simulink model "mat_ffun"  (R2015b)
settings: Solver=VariableStepAuto  StartTime=0.0  StopTime=100  RelTol=1e-3
undefined symbols (not defined in the file): alpha, delta_e, V, w
settings Model: Creator=Pramod  LastModifiedBy=Pramod

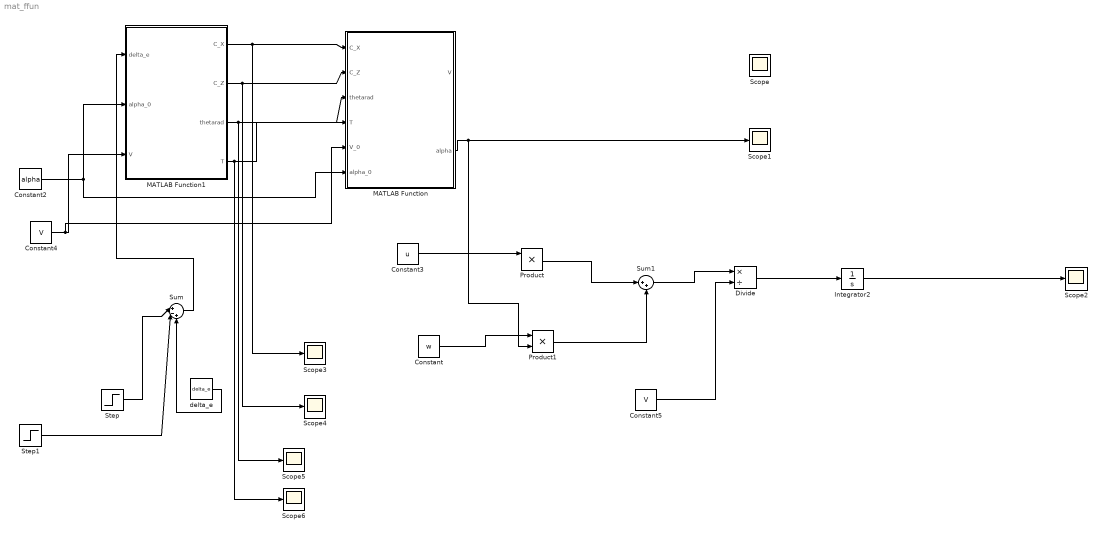
== system mat_ffun ==
  Constant : Constant  Value=w
  Constant2 : Constant  Value=alpha
  Constant3 : Constant  Value=u
  Constant4 : Constant  Value=V
  Constant5 : Constant  Value=V
  Divide : Product  Inputs=*/
  Integrator2 : Integrator  InitialCondition=V
  MATLAB Function : MATLAB Function  TreatAsAtomicUnit=on
  MATLAB Function1 : MATLAB Function  TreatAsAtomicUnit=on
  Product : Product
  Product1 : Product
  Scope{,1..6} (7 alike) : Scope
  Step : Step  Time=55  After=pi/180  SampleTime=0
  Step1 : Step  Time=95  After=pi/180  SampleTime=0
  Sum : Sum  Inputs=|+-+
  Sum1 : Sum  Inputs=|++
  delta_e : Constant  Value=delta_e
  wires:
  Constant2/1 -> MATLAB Function1/2(alpha_0), MATLAB Function/6(alpha_0)
  MATLAB Function1/1(C_X) -> Scope3/1, MATLAB Function/1(C_X)
  MATLAB Function1/2(C_Z) -> Scope4/1, MATLAB Function/2(C_Z)
  MATLAB Function1/3(thetarad) -> Scope5/1, MATLAB Function/3(thetarad)
  ? -> Scope/1, Product/2
  MATLAB Function/2(alpha) -> Product1/2, Scope1/1
  MATLAB Function1/4(T) -> Scope6/1, MATLAB Function/4(T)
  Step/1 -> Sum/1
  Step1/1 -> Sum/2
  Constant3/1 -> Product/1
  Constant/1 -> Product1/1
  Product/1 -> Sum1/1
  Product1/1 -> Sum1/2
  Sum1/1 -> Divide/1
  Constant5/1 -> Divide/2
  Divide/1 -> Integrator2/1
  Integrator2/1 -> Scope2/1
  Constant4/1 -> MATLAB Function/5(V_0), MATLAB Function1/3(V)
  delta_e/1 -> Sum/3
  Sum/1 -> MATLAB Function1/1(delta_e)

== matlab function mat_ffun/MATLAB Function1 ==
  data: delta_e input; alpha_0 input; C_X output; C_Z output; thetarad output; T output; V input
function [C_X,C_Z,thetarad,T] = fcn(delta_e,alpha_0,V)
% delta_e=u(1);
% T=u(2);
% alpha=u(3);
 alpharad=alpha_0*pi/180;
g = 9.8;
rho = 1.225;
q=0
m = 1043.26;
C_bar = 1.493;
b = 10.911;
S_ref = 16.1651;


C_L_0 = 0.25;
C_L_alpha = 4.47;
C_L_q = 1.7;
C_L_delta_e = 0.3476;

% Ignore all other C_D derivatives excluding C_D_0
% Use C_D = C_D_0 + k*C_L^2

C_D_0 = 0.036;
k = 0.3;

C_Y_beta = -0.31;
C_Y_p = -0.037;
C_Y_r = 0.21;
C_Y_delta_a = 0;

C_l_beta = -0.089;
C_l_p = -0.47;
C_l_r = 0.096;
C_l_delta_a = -0.09;
C_l_delta_r = 0.0147;

C_M_0 = -0.02;
C_M_alpha = -1.8;
C_M_alpha_dot = -12.4;
C_M_delta_e = -1.28;

C_N_beta = 0.065;
C_N_p = -0.03;
C_N_r = -0.99;
C_N_delta_a = -0.0053;
C_N_delta_r = -0.0657;
C_L = C_L_0 + C_L_alpha*alpharad +   C_L_delta_e*delta_e
C_D = C_D_0 + k*C_L^2;
C_X = -C_D*cos(alpharad) + C_L*sin(alpharad);
C_Z = -C_D*sin(alpharad) - C_L*cos(alpharad);
cns=-rho*V^2*S_ref*C_Z/(2*m*g);
thetarad=acos(cns);
T=m*g*sin(thetarad)-(rho*S_ref*C_X*V^2)/2
% y(1)=C_L;
% y(2)=C_D;
% y(3)=C_X;
% y(4)=C_Z;

== matlab function mat_ffun/MATLAB Function ==
  data: V output; C_X input; C_Z input; thetarad input; T input; alpha output; V_0 input; alpha_0 input
function [V,alpha] = fcn(C_X,C_Z,thetarad,T,V_0,alpha_0 )
g = 9.8;
rho = 1.225;
q=0
m = 1043.26;
% C_bar = 1.493;
% b = 10.911;
 S_ref = 16.1651;
u=sqrt(V_0^2/(sec(alpharad)*sec(alpharad)));
w=sqrt(V^2-u^2);
% 
% C_L_0 = 0.25;
% C_L_alpha = 4.47;
% C_L_q = 1.7;
% C_L_delta_e = 0.3476;
% 
% % Ignore all other C_D derivatives excluding C_D_0
% % Use C_D = C_D_0 + k*C_L^2
% 
% C_D_0 = 0.036;
% k = 0.3;
% 
% C_Y_beta = -0.31;
% C_Y_p = -0.037;
% C_Y_r = 0.21;
% C_Y_delta_a = 0;
% 
% C_l_beta = -0.089;
% C_l_p = -0.47;
% C_l_r = 0.096;
% C_l_delta_a = -0.09;
% C_l_delta_r = 0.0147;
% 
% C_M_0 = -0.02;
% C_M_alpha = -1.8;
% C_M_alpha_dot = -12.4;
% C_M_delta_e = -1.28;
% 
% C_N_beta = 0.065;
% C_N_p = -0.03;
% C_N_r = -0.99;
% C_N_delta_a = -0.0053;
% C_N_delta_r = -0.0657;
% C_L = C_L_0 + C_L_alpha*alpharad +   C_L_delta_e*delta_e
% C_D = C_D_0 + k*C_L^2;
% C_X = -C_D*cos(alpharad) + C_L*sin(alpharad);
% C_Z = -C_D*sin(alpharad) - C_L*cos(alpharad);
% u=sqrt(V^2/(sec(alpha*pi/180)*sec(alpha*pi/180)));
% w=sqrt(V^2-u^2);
udot=T/m-g*sin(thetarad)+(0.5*rho*V^2*S_ref*C_X/m)
wdot=(0.5*rho*V^2*S_ref*C_Z/m)+g*cos(thetarad)

Vdot=(u*udot+w*wdot)/V
alphadot=(u*wdot-w*udot)/V
llong=@(t,y)[Vdot;alphadot];
y0=[V alpha];

[t2,y2]=ode45(llong,[110 300],y0)
